simulink model "ME4391L_Goulenko_Lab2_Problem4"  (R2023a)
settings: Solver=VariableStepAuto  StartTime=0.0  StopTime=10.0  RelTol=1e-3
settings Model: Creator=Gregory  LastModifiedBy=Gregory

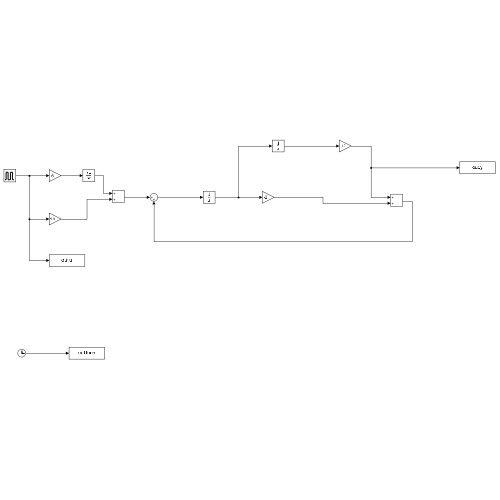
[thumbnail: Simulink's stored preview of the top-level diagram]
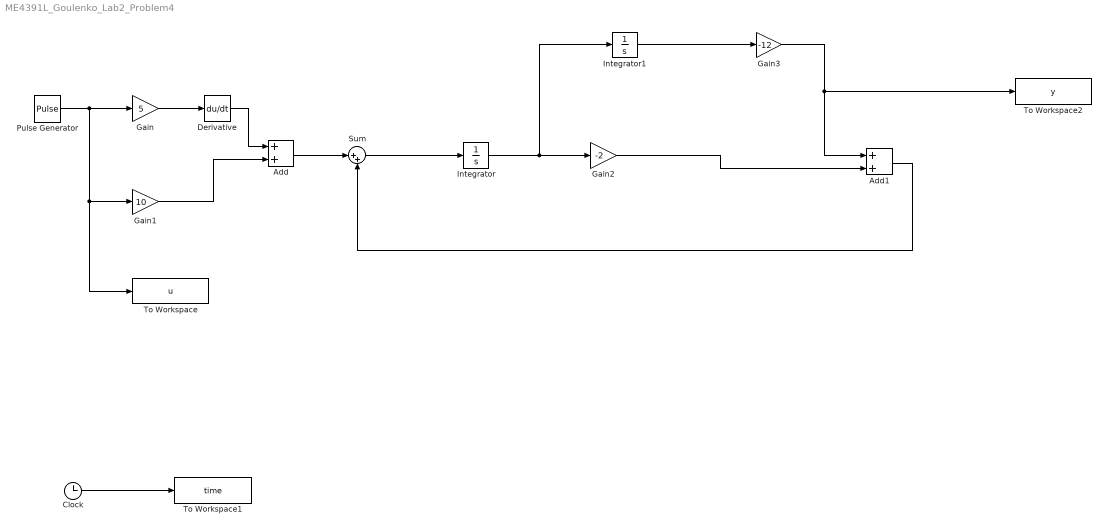
== system ME4391L_Goulenko_Lab2_Problem4 ==
  Add : Sum
  Add1 : Sum
  Clock : Clock
  Derivative : Derivative
  Gain : Gain  Gain=5
  Gain1 : Gain  Gain=10
  Gain2 : Gain  Gain=-2
  Gain3 : Gain  Gain=-12
  Integrator : Integrator
  Integrator1 : Integrator
  Pulse Generator : DiscretePulseGenerator  PulseType=Time based  Amplitude=10  Period=20  PulseWidth=50
  Sum : Sum  Inputs=|++
  To Workspace : ToWorkspace  VariableName=u  SaveFormat=Timeseries  SampleTime=-1
  To Workspace1 : ToWorkspace  VariableName=time  SaveFormat=Timeseries  SampleTime=-1
  To Workspace2 : ToWorkspace  VariableName=y  SaveFormat=Timeseries  SampleTime=-1
  wires:
  Pulse Generator/1 -> Gain/1, To Workspace/1, Gain1/1
  Gain/1 -> Derivative/1
  Gain1/1 -> Add/2
  Derivative/1 -> Add/1
  Add/1 -> Sum/1
  Clock/1 -> To Workspace1/1
  Sum/1 -> Integrator/1
  Integrator/1 -> Integrator1/1, Gain2/1
  Integrator1/1 -> Gain3/1
  Gain3/1 -> To Workspace2/1, Add1/1
  Gain2/1 -> Add1/2
  Add1/1 -> Sum/2
